simulink model "Model_will_test"  (R2025b)
settings: Solver=VariableStepAuto  StartTime=0.0  StopTime=35  RelTol=1e-2  AbsTol=1e-2  EnableMultiTasking=on
values from neighbouring files (symbols this model uses):
  Ad = sysd.A    [MARLUP_FINAL.m]    (also in marlup_params.mat = [1 0 0 0 0 0 0.01 1 0 0 0 0 ... (36 elements, 6x6)]; test.m)
  Bd = sysd.B    [MARLUP_FINAL.m]    (also in marlup_params.mat = [8.07172860911e-06 0.00161434572182 0 0 0 0 0 0 8.0717286091; test.m)
  C = [1 0 0 0 0 0 ... (first row only)    [MARLUP_FINAL.m]    (also in marlup_identify.m = [1 0 0 0 0 0; 0 0 1 0 0 0; 0 0 0 0 1 0]; marlup_params.mat = [1 0 0 0 0 0 0 1 0 0 0 0 ... (18 elements, 3x6)]; script_will.m; script_will_corregido.m)
  Cd = sysd.C    [MARLUP_FINAL.m]    (also in marlup_params.mat = [1 0 0 0 0 0 0 1 0 0 0 0 ... (18 elements, 3x6)]; test.m)
  Dd = sysd.D    [MARLUP_FINAL.m]    (also in marlup_params.mat = [0  0  0; 0  0  0; 0  0  0]; test.m)
  F_grav = [435.215309817 435.215309817 435.215309817]    [marlup_params.mat]    (also in script_will_corregido.m = T \ [0; 0; M*g])
  F_sat = 8000    [marlup_params.mat]    (also in script_will_corregido.m)
  Ki = [-334.50084  1.1108667168e-12  -7.58489313833e-13; -7.0645634967e-14  -334.50084  -2.5694260705e-12; -1.41673451802e-12  -1.16842800425e-12  -3656.258838]    [marlup_params.mat]    (also in script_will.m = Ka(:, n+1:end); script_will_corregido.m = Ka(:, n+1:end); script_will_old.m = Ka(:, n+1:end); script_will_posicion.m = Ka(:, n+1:end))
  Kx = [308.336131576 -8.19268492329e-14 1.78801149562e-12 67.7754953843 -1.07383820994e-13 5.13036333214e-13 -5.85790721927e-13 308.336131576 7.47314391083e-13 -1.51788465993e-13 67.7754953843 1.74261406414e-13 ... (18 elements, 3x6)]    [marlup_params.mat]    (also in script_will.m = Ka(:, 1:n); script_will_corregido.m = Ka(:, 1:n); script_will_old.m = Ka(:, 1:n); script_will_posicion.m = Ka(:, 1:n))
  m = t > tskip & t <= tfit    [marlup_identify.m]    (also in marlup_params.mat = 3; script_will.m = size(B,2); script_will_corregido.m = 3; script_will_old.m = size(B,2))
  N = zeros(size(Gw,2), p)    [script_will.m]    (also in script_will_old.m = zeros(6,3))
  P_reorder = [0  0  1; 0  1  0; 1  0  0]    [marlup_params.mat]    (also in script_will.m = [0 0 1; script_will_corregido.m = [0 0 1; script_will_old.m = [0 0 1)
  ref_heave = 0.1    [marlup_params.mat]    (also in script_will_corregido.m)
  ref_pitch = 0    [marlup_params.mat]    (also in script_will_corregido.m)
  ref_roll = 0    [marlup_params.mat]    (also in script_will_corregido.m)
  Rv = [7.61543549467e-05  0  0; 0  7.61543549467e-05  0; 0  0  9e-06]    [marlup_params.mat]    (also in script_will_corregido.m = diag([(0.5*pi/180)^2, (0.5*pi/180)^2, (3e-3)^2]))
  Tinv = [-1.00804199915  -1.74597995868  0.655227299445; 2.01608399829  1.95401598016e-16  0.655227299445; -1.00804199915  1.74597995868  0.655227299445]    [marlup_params.mat]    (also in script_will.m = pinv(T); script_will_corregido.m = inv(T); script_will_old.m = pinv(T); tests_will.m = inv(T))
  Ts = 0.01    [MARLUP_FINAL.m]    (also in marlup_params.mat; script_will.m; script_will_corregido.m; script_will_old.m)
  xi_max = [7.90847766797 6.84894256573 1.6696716551]    [marlup_params.mat]    (also in script_will_corregido.m = abs(Ki) \ (umax*0.8))
  Z = squeeze(lg.getElement('Z').Values.Data)    [test.m]
undefined symbols (not defined in the file or in its folder): DiscIntNeverNeededParam, Discrete, Time, X, Y
libraries: sm_lib x72, nesl_utility x9, ctrlSharedLib x1
(part 4 of 4)

== matlab function Model_will_test/P-M SPECTRUM/P-M SPECTRUM ==
  settings: updateMethod=DISCRETE
  data: t input; heave output; Hs input; Tp input; pitch output; roll output
function [heave, pitch, roll] = fcn(t, Hs, Tp)
%#codegen
% Esta función genera la elevación (heave), y los ángulos de inclinación 
% (pitch y roll) en el origen (0,0) para un oleaje P-M.
%
% Se utiliza t==0 para una inicialización robusta.

% -- Declaración de variables persistentes --
% Estas variables retienen su valor entre llamadas a la función.
persistent Anm fase omega kx ky

% -- Bloque de Inicialización --
% Este código se ejecuta UNA SOLA VEZ, al puro inicio de la simulación (t=0).
if t == 0
    
    % Parámetros fijos de la simulación
    N = 100;         % Número de componentes de frecuencia
    M = 50;          % Número de componentes de dirección
    g = 9.81;        % Aceleración de la gravedad

    % --- PRE-CÁLCULOS (se ejecutan solo una vez) ---
    fp = 1 / Tp;
    f_max = 4 * fp;
    df = f_max / N;
    f = df:df:f_max;
    omega = 2 * pi * f;

    d_theta = 2*pi / M;
    theta = d_theta:d_theta:2*pi;
    
    % Semilla fija: el mismo estado de mar en cada corrida, para poder
    % comparar controladores y reproducir resultados.
    rng(42);

    % Generar fases aleatorias (fijas para toda la simulación)
    fase = 2 * pi * rand(N, M);

    k_o = omega.^2 / g;
    kx = k_o' * cos(theta);
    ky = k_o' * sin(theta);
    
    A_pm = (5/16) * Hs^2 * fp^4;
    S = (A_pm ./ f.^5) .* exp(-1.25 * (fp^4 ./ f.^4));

    s = 10;
    D_theta = (2/pi) * (cos(theta/2)).^(2*s);
    D_theta(theta < -pi/2 | theta > pi/2) = 0;
    
    Anm = sqrt(2 * S' .* D_theta * df * d_theta);
end

% -- CÁLCULOS EN CADA PASO DE TIEMPO --
% Se requiere que las variables persistentes no estén vacías después de t=0
if isempty(Anm)
    % Si la inicialización no ha ocurrido (ej. si la simulación no empezó en t=0),
    % se asignan salidas cero para evitar errores.
    heave = 0;
    pitch = 0;
    roll = 0;
else
    % Cálculos normales para t > 0
    arg = -omega' * t + fase;
    heave = sum(Anm .* cos(arg), 'all');
    d_etadx = sum(Anm .* kx .* sin(arg), 'all');
    d_etady = sum(Anm .* ky .* sin(arg), 'all');
    pitch = atan(d_etadx);
    roll  = atan(d_etady);
end

end
